simulink model "GotoFromEx"  (Simulink 6.3)
settings: Solver=VariableStepDiscrete  StartTime=0.0  StopTime=10.0  RelTol=1e-3
InitFcn:
  | %% DSPBuilder Start
  | alt_dspbuilder_update_model(bdroot)
  | %% DSPBuilder End
libraries: allblocks_alteradspbuilder2 x22
settings Model: Creator=gnixon  LastModifiedBy=delphick
settings OptimizationCC: BooleanDataType=off  InlineInvariantSignals=on
settings DebuggingCC: SolverPrmCheckMsg=none
settings HardwareCC: TargetUnknown=on

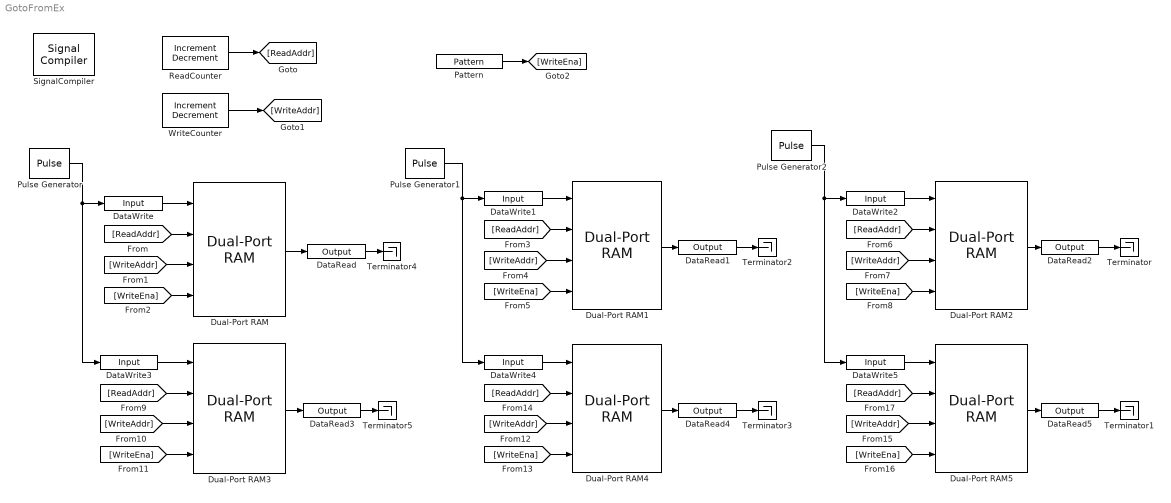
== system GotoFromEx ==
  DataRead : allblocks_alteradspbuilder2/Output  iofile=C:\workspace_clean\Documentation\DesignExamples\Tutorials\UsingFromGoto\tb_GotoFromEx\GotoFromEx_DataRead.capture  BusType=Signed Integer  bwl=8  bwr=8  PORTTYPE=Output
  DataRead1 : allblocks_alteradspbuilder2/Output  iofile=C:\workspace_clean\Documentation\DesignExamples\Tutorials\UsingFromGoto\tb_GotoFromEx\GotoFromEx_DataRead1.capture  BusType=Signed Integer  bwl=8  bwr=8  PORTTYPE=Output
  DataRead2 : allblocks_alteradspbuilder2/Output  iofile=C:\workspace_clean\Documentation\DesignExamples\Tutorials\UsingFromGoto\tb_GotoFromEx\GotoFromEx_DataRead2.capture  BusType=Signed Integer  bwl=8  bwr=8  PORTTYPE=Output
  DataRead3 : allblocks_alteradspbuilder2/Output  iofile=C:\workspace_clean\Documentation\DesignExamples\Tutorials\UsingFromGoto\tb_GotoFromEx\GotoFromEx_DataRead3.capture  BusType=Signed Integer  bwl=8  bwr=8  PORTTYPE=Output
  DataRead4 : allblocks_alteradspbuilder2/Output  iofile=C:\workspace_clean\Documentation\DesignExamples\Tutorials\UsingFromGoto\tb_GotoFromEx\GotoFromEx_DataRead4.capture  BusType=Signed Integer  bwl=8  bwr=8  PORTTYPE=Output
  DataRead5 : allblocks_alteradspbuilder2/Output  iofile=C:\workspace_clean\Documentation\DesignExamples\Tutorials\UsingFromGoto\tb_GotoFromEx\GotoFromEx_DataRead5.capture  BusType=Signed Integer  bwl=8  bwr=8  PORTTYPE=Output
  DataWrite : allblocks_alteradspbuilder2/Input  iofile=C:\workspace_clean\Documentation\DesignExamples\Tutorials\UsingFromGoto\tb_GotoFromEx\GotoFromEx_DataWrite.salt  BusType=Signed Integer  bwl=8  bwr=8  SpecifyClock=off  PORTTYPE=Input
  DataWrite1 : allblocks_alteradspbuilder2/Input  iofile=C:\workspace_clean\Documentation\DesignExamples\Tutorials\UsingFromGoto\tb_GotoFromEx\GotoFromEx_DataWrite1.salt  BusType=Signed Integer  bwl=8  bwr=8  SpecifyClock=off  PORTTYPE=Input
  DataWrite2 : allblocks_alteradspbuilder2/Input  iofile=C:\workspace_clean\Documentation\DesignExamples\Tutorials\UsingFromGoto\tb_GotoFromEx\GotoFromEx_DataWrite2.salt  BusType=Signed Integer  bwl=8  bwr=8  SpecifyClock=off  PORTTYPE=Input
  DataWrite3 : allblocks_alteradspbuilder2/Input  iofile=C:\workspace_clean\Documentation\DesignExamples\Tutorials\UsingFromGoto\tb_GotoFromEx\GotoFromEx_DataWrite3.salt  BusType=Signed Integer  bwl=8  bwr=8  SpecifyClock=off  PORTTYPE=Input
  DataWrite4 : allblocks_alteradspbuilder2/Input  iofile=C:\workspace_clean\Documentation\DesignExamples\Tutorials\UsingFromGoto\tb_GotoFromEx\GotoFromEx_DataWrite4.salt  BusType=Signed Integer  bwl=8  bwr=8  SpecifyClock=off  PORTTYPE=Input
  DataWrite5 : allblocks_alteradspbuilder2/Input  iofile=C:\workspace_clean\Documentation\DesignExamples\Tutorials\UsingFromGoto\tb_GotoFromEx\GotoFromEx_DataWrite5.salt  BusType=Signed Integer  bwl=8  bwr=8  SpecifyClock=off  PORTTYPE=Input
  Dual-Port RAM{,1..5} (6 alike) : allblocks_alteradspbuilder2/Dual-Port RAM  numwords=2^(7)  BusType=Inferred  bwl=8  bwr=0  memory_type=AUTO  ram_type=DualRAM  initialization=Blank  init_file=input.hex  init_array=[0:1:15]  register_outputs=off  use_ena=off  ClockPhase=1
  Pattern : allblocks_alteradspbuilder2/Pattern  Sequence=100000  SpecifyClock=off  use_ena=off  use_sclr=off
  Pulse Generator : DiscretePulseGenerator  PulseType=Time based  PulseWidth=50
  Pulse Generator1 : DiscretePulseGenerator  PulseType=Time based  PulseWidth=50
  Pulse Generator2 : DiscretePulseGenerator  PulseType=Time based  PulseWidth=50
  ReadCounter : allblocks_alteradspbuilder2/Increment Decrement  BusType=Signed Integer  bwl=8  bwr=0  SpecifyClock=off  clr_value=0  direction=Increment  phase_selection=1  use_ena=off  use_sclr=off
  SignalCompiler : allblocks_alteradspbuilder2/Signal Compiler  DeviceFamily=Stratix IV  DeviceName=AUTO  EnableSignalTap=off  SignalTapDepth=128  UseBoardBlock=off  StpUseDefaultClock=on  StpClock=clock
  Terminator{,1..5} (6 alike) : Terminator
  WriteCounter : allblocks_alteradspbuilder2/Increment Decrement  BusType=Signed Integer  bwl=8  bwr=0  SpecifyClock=off  clr_value=0  direction=Increment  phase_selection=1  use_ena=off  use_sclr=off
  wires:
  DataWrite/1 -> Dual-Port RAM/1
  Dual-Port RAM/1 -> DataRead/1
  [ReadAddr] -> Dual-Port RAM/2
  [WriteAddr] -> Dual-Port RAM/3
  [WriteEna] -> Dual-Port RAM/4
  DataWrite1/1 -> Dual-Port RAM1/1
  Dual-Port RAM1/1 -> DataRead1/1
  [ReadAddr] -> Dual-Port RAM1/2
  [WriteAddr] -> Dual-Port RAM1/3
  [WriteEna] -> Dual-Port RAM1/4
  DataWrite2/1 -> Dual-Port RAM2/1
  Dual-Port RAM2/1 -> DataRead2/1
  [ReadAddr] -> Dual-Port RAM2/2
  [WriteAddr] -> Dual-Port RAM2/3
  [WriteEna] -> Dual-Port RAM2/4
  DataWrite3/1 -> Dual-Port RAM3/1
  Dual-Port RAM3/1 -> DataRead3/1
  [ReadAddr] -> Dual-Port RAM3/2
  [WriteAddr] -> Dual-Port RAM3/3
  [WriteEna] -> Dual-Port RAM3/4
  DataWrite4/1 -> Dual-Port RAM4/1
  Dual-Port RAM4/1 -> DataRead4/1
  [ReadAddr] -> Dual-Port RAM4/2
  [WriteAddr] -> Dual-Port RAM4/3
  [WriteEna] -> Dual-Port RAM4/4
  DataWrite5/1 -> Dual-Port RAM5/1
  Dual-Port RAM5/1 -> DataRead5/1
  [ReadAddr] -> Dual-Port RAM5/2
  [WriteAddr] -> Dual-Port RAM5/3
  [WriteEna] -> Dual-Port RAM5/4
  ReadCounter/1 -> [ReadAddr]
  WriteCounter/1 -> [WriteAddr]
  Pattern/1 -> [WriteEna]
  DataRead2/1 -> Terminator/1
  DataRead5/1 -> Terminator1/1
  DataRead1/1 -> Terminator2/1
  DataRead4/1 -> Terminator3/1
  DataRead/1 -> Terminator4/1
  DataRead3/1 -> Terminator5/1
  Pulse Generator/1 -> DataWrite/1, DataWrite3/1
  Pulse Generator1/1 -> DataWrite1/1, DataWrite4/1
  Pulse Generator2/1 -> DataWrite2/1, DataWrite5/1
